simulink model "A3_A4_2"  (R2017a)
settings: Solver=VariableStepAuto  StartTime=0.00001  StopTime=0.02  MaxStep=1e-4  RelTol=1e-3
libraries: powerlib x11, powerlib_meascontrol x2
settings Model: Creator=Amir Reza  LastModifiedBy=Amir Reza

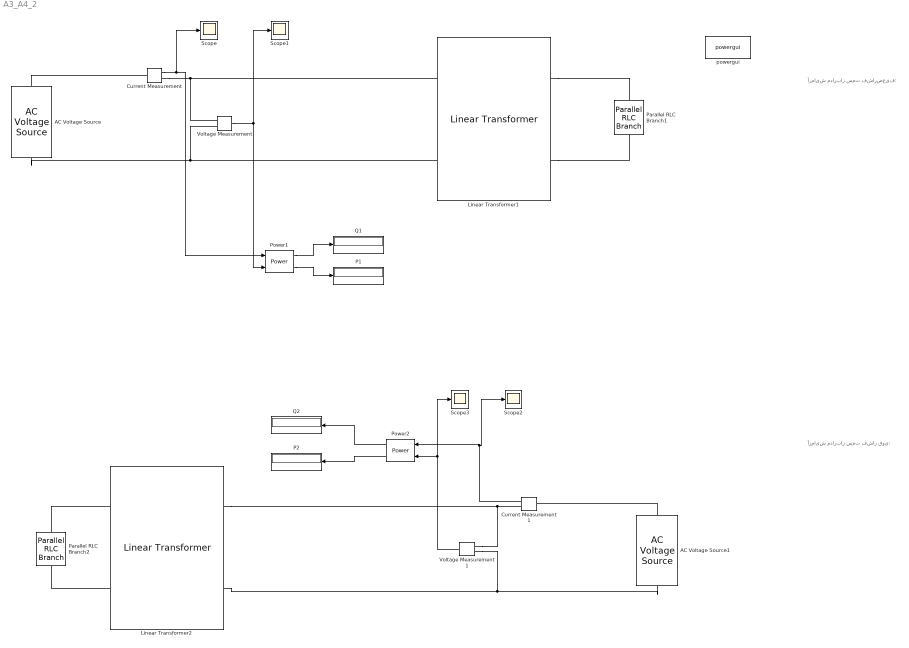
== system A3_A4_2 ==
  note: آزمایش مدارباز سمت فشارضعیف:
  note: آزمایش مدارباز سمت فشار قوی:
  AC Voltage Source : powerlib/Electrical Sources/AC Voltage Source  Amplitude=240  Phase=0  Frequency=50  SampleTime=0  Measurements=None  BusType=swing  Pref=10e3  Qref=0  Qmin=-inf  Qmax=+inf
  AC Voltage Source1 : powerlib/Electrical Sources/AC Voltage Source  Amplitude=2400  Phase=0  Frequency=50  SampleTime=0  Measurements=None  BusType=swing  Pref=10e3  Qref=0  Qmin=-inf  Qmax=+inf
  Current Measurement : powerlib/Measurements/Current Measurement  PhasorSimulation=off  OutputType=Complex  PSBequivalent=0
  Current Measurement1 : powerlib/Measurements/Current Measurement  PhasorSimulation=off  OutputType=Complex  PSBequivalent=0
  Linear Transformer1 : powerlib/Elements/Linear Transformer  UNITS=SI  NominalPower=[75e3 50 ]  winding1=[240 6e-3 7.57e-5]  winding2=[2400 0.23 9.74e-3]  ThreeWindings=off  winding3=[3.15e+05 1.0502e+06 354.69]  RmLm=[25 3.97e-2]  Measurements=None  DataType=on
  Linear Transformer2 : powerlib/Elements/Linear Transformer  UNITS=SI  NominalPower=[75e3 50 ]  winding1=[240 6e-3 7.57e-5]  winding2=[2400 0.23 9.74e-3]  ThreeWindings=off  winding3=[3.15e+05 1.0502e+06 354.69]  RmLm=[25 3.97e-2]  Measurements=None  DataType=on
  P1 : Display
  P2 : Display
  Parallel RLC Branch1 : powerlib/Elements/Parallel RLC Branch  LConnTagsString=a  RConnTagsString=__new0  BranchType=R  Resistance=1e6  Inductance=1e-3  SetiL0=off  InitialCurrent=0  Capacitance=1e-6  Setx0=off  InitialVoltage=0  Measurements=None
  Parallel RLC Branch2 : powerlib/Elements/Parallel RLC Branch  LConnTagsString=a  RConnTagsString=__new0  BranchType=R  Resistance=1e6  Inductance=1e-3  SetiL0=off  InitialCurrent=0  Capacitance=1e-6  Setx0=off  InitialVoltage=0  Measurements=None
  Power1 : powerlib_meascontrol/Measurements/Power  Freq=50  Vinit=[1, 0]  Iinit=[1, 0]  Ts=0
      settings: SourceProductName=Simscape Power Systems
  Power2 : powerlib_meascontrol/Measurements/Power  Freq=50  Vinit=[1, 0]  Iinit=[1, 0]  Ts=0
      settings: SourceProductName=Simscape Power Systems
  Q1 : Display
  Q2 : Display
  Scope{,1..3} (4 alike) : Scope
  Voltage Measurement : powerlib/Measurements/Voltage Measurement  PhasorSimulation=off  OutputType=Complex  PSBequivalent=0
  Voltage Measurement1 : powerlib/Measurements/Voltage Measurement  PhasorSimulation=off  OutputType=Complex  PSBequivalent=0
  powergui : powerlib/powergui  Priority=1  SimulationMode=Continuous  SampleTime=50e-6  frequency=50  Iterations=50  frequencyindice=50  Pbase=100e6  ErrMax=1e-4  UnitsV=kV  UnitsW=MW  buscounter=0  FunctionMessages=off  echomessages=off  EnableUseOfTLC=off  CurrentSourceSwitches=off  DisableSnubberDevices=off  DisableRonSwitches=off  DisableVfSwitches=off  DisplayEquations=off  SolverType=Tustin/Backward Euler (TBE)  Interpol=off  ExternalGateDelay=off  methode=off  Ts=100  x0status=blocks  SPID=on  SwTol=0  HookPort=off  RestoreLinks=warning  ResistiveCurrentMeasurement=off  Frange=[-50:50]  Ylog=off  Xlog=off  ShowGrid=off  save=off  variable=ZData  structure=0  ZoomFFT=off  StartTime=0.0  cycles=1  DisplayStyle=1  fundamental=60  FreqAxis=off  MaxFrequency=1000  frequencyindicesteady=50  RmsSteady=1  display=off
  wires:
  Power1/1 -> P1/1
  Power1/2 -> Q1/1
  Current Measurement/1 -> Scope/1, Power1/2
  Voltage Measurement/1 -> Scope1/1, Power1/1
  Voltage Measurement1/1 -> Scope3/1, Power2/1
  Current Measurement1/1 -> Scope2/1, Power2/2
  Power2/1 -> P2/1
  Power2/2 -> Q2/1
  connections:
  Current Measurement/LConn1 -- AC Voltage Source/RConn1
  Current Measurement/RConn1 -- Linear Transformer1/LConn1 -- Voltage Measurement/LConn1
  AC Voltage Source/LConn1 -- Linear Transformer1/LConn2 -- Voltage Measurement/LConn2
  Linear Transformer1/RConn2 -- Parallel RLC Branch1/RConn1
  Linear Transformer1/RConn1 -- Parallel RLC Branch1/LConn1
  Linear Transformer2/LConn1 -- Parallel RLC Branch2/LConn1
  Linear Transformer2/LConn2 -- Parallel RLC Branch2/RConn1
  AC Voltage Source1/RConn1 -- Current Measurement1/LConn1
  Current Measurement1/RConn1 -- Voltage Measurement1/LConn1 -- Linear Transformer2/RConn1
  AC Voltage Source1/LConn1 -- Voltage Measurement1/LConn2 -- Linear Transformer2/RConn2
